simulink model "no3_PI_Controller"  (R2025a)
settings: Solver=FixedStepAuto  StartTime=0.0  StopTime=50  FixedStep=0.2  RelTol=1e-3
libraries: simulink x1
settings Model: Creator=ayeo  LastModifiedBy=ayeo

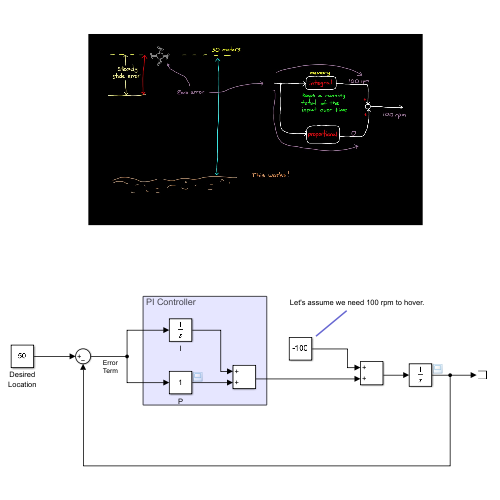
[thumbnail: Simulink's stored preview of the top-level diagram]
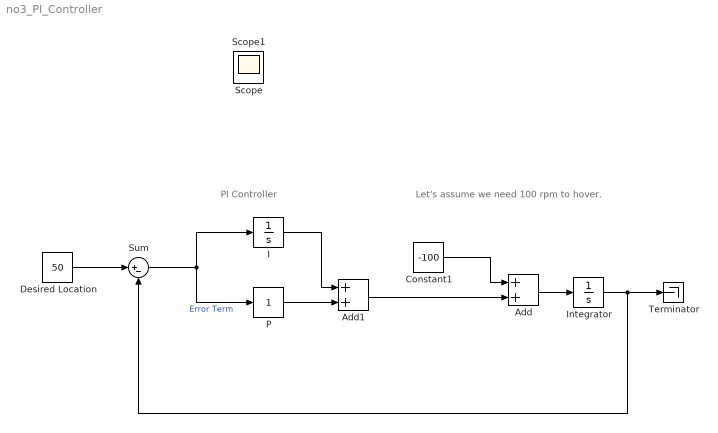
== system no3_PI_Controller ==
  note: Let's assume we need 100 rpm to hover.
  note: PI Controller
  Add : Sum
  Add1 : Sum
  Constant1 : Constant  Value=-100
  Desired Location : Constant  Value=50
  I : Integrator
  Integrator : Integrator
  P : simulink/Math Operations/Slider Gain  gain=1  low=0.1  high=100
  Sum : Sum  Inputs=|+-
  Terminator : Terminator
  Scope : Scope
      settings: ActiveDisplayYMinimum=-52.467199180125249  ActiveDisplayYMaximum=86.081205775591656
  Scope1 : Scope
      settings: ActiveDisplayYMinimum=81.26535  ActiveDisplayYMaximum=268.74829
  wires:
  Desired Location/1 -> Sum/1
  Integrator/1 -> Sum/2, Terminator/1
  Add/1 -> Integrator/1
  Constant1/1 -> Add/1
  Add1/1 -> Add/2
  I/1 -> Add1/1
  Sum/1 -> I/1, P/1  "Error Term"
  P/1 -> Add1/2
